simulink model "System_model_discrete"  (R2022a)
settings: Solver=FixedStepDiscrete  StartTime=0.0  StopTime=T_final  FixedStep=T_sample  RelTol=1e-3
values from neighbouring files (symbols this model uses):
  A_bar_d = readmatrix('A_bar_d.csv')    [Run_model_WDS.m]
  B_bar_d = readmatrix('B_bar_d.csv')    [Run_model_WDS.m]
  BDD_thresh = 5    [Run_model_WDS.m]    (also in run_model.m = 0.05)
  C_obsv_d = readmatrix('C_obsv_d.csv')    [Run_model_WDS.m]    (also in run_model.m = C_obsv; run_model_power_system.m = C_obsv)
  D_obsv_d = readmatrix('D_obsv_d.csv')    [Run_model_WDS.m]    (also in run_model.m = D_obsv; run_model_power_system.m = D_obsv)
  l = n_meas    [run_model.m]
  L_obsv = place(A_bar_d.',C_obsv_d.',P).'    [run_model.m]    (also in run_model_power_system.m)
  load_buses = [zeros(n_gen,1); ones(n_bus-n_gen,1)]    [run_model.m]    (also in run_model_power_system.m)
  m = n_meas    [run_model.m]
  max_attack = 1000    [Run_model_WDS.m]
  n = n_states    [run_model.m]
  n_attack = round(attack_percentage*n_meas)    [Run_model_WDS.m]    (also in run_model.m = round(0.2*n_meas))
  n_bus = size(bus,1)    [run_model.m]    (also in run_model_power_system.m)
  n_gen = size(gen,1)    [run_model.m]    (also in run_model_power_system.m)
  n_meas = size(C_obsv_d,1)    [Run_model_WDS.m]    (also in run_model.m = n_gen + n_bus; run_model_power_system.m = n_gen + n_bus)
  n_states = 2*n_gen    [run_model.m]    (also in run_model_power_system.m)
  q0 = ones(m,T)    [run_model.m]
  r_tau = chi2inv(0.1,n_meas)    [Run_model_WDS.m]
  Sigma = diag(sigma)    [Run_model_WDS.m]    (also in run_model.m)
  sigma_inv_k = 1e2*(3 + 2*rand(n_meas,1))    [Run_model_WDS.m]    (also in run_model.m = 1e4*(3 + 2*rand(m,1)); sigma_inv_k.mat = [541957.05841 17086.3156535 20847.4062112 958.936090052 8825)
  Sigma_inv_k = diag(sigma_inv_k)    [Run_model_WDS.m]    (also in run_model.m)
  T = round(2*n_states)    [Run_model_WDS.m]    (also in run_model.m = round(2*n); run_model_power_system.m = 10)
  T_sample = 0.01    [Run_model_WDS.m]    (also in run_model.m; run_model_power_system.m)
  T_start_attack = 0.1*T_final    (= 0.8)    [Run_model_WDS.m]    (also in run_model.m = 1.6; run_model_power_system.m)
  U0 = zeros(n_int,T+1)    [Run_model_WDS.m]    (also in run_model.m = zeros(m,T); run_model_power_system.m)
  x0 = zeros(n_states,1)    [Run_model_WDS.m]    (also in run_model.m; run_model_power_system.m)
  Y0 = zeros(n_meas,T)    [Run_model_WDS.m]    (also in run_model.m = zeros(m,T); run_model_power_system.m)
undefined symbols (not defined in the file or in its folder): G_T, HT, PhiT, sigbuilder_block, T_start_opt, Theta_T
libraries: simulink x5
settings Model: Creator=oanubi  LastModifiedBy=Abelb
settings SolverCC: AlgebraicLoopSolver=TrustRegion
settings DebuggingCC: UnconnectedInputMsg=warning  UnconnectedOutputMsg=warning  UnconnectedLineMsg=warning  SFMachineParentedDataDiag=warning

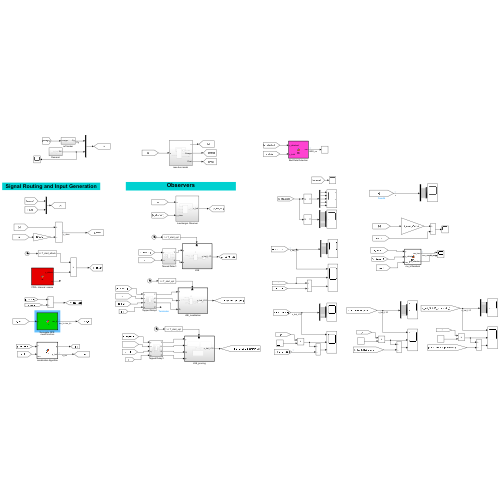
[thumbnail: Simulink's stored preview of the top-level diagram]
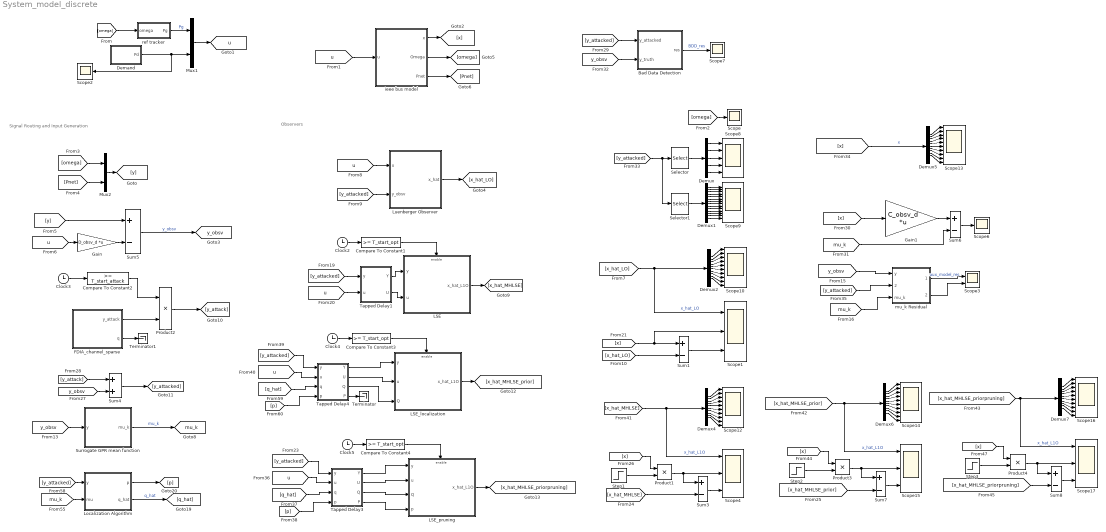
== system System_model_discrete ==
  note: Observers
  note: Signal Routing and Input Generation
  Bad Data Detection : MATLAB Function  TreatAsAtomicUnit=on
  Clock{2..5} (4 alike) : Clock
  Compare To Constant1 : simulink/Logic and Bit Operations/Compare To Constant  relop=>=  const=T_start_opt  OutDataTypeStr=boolean
  Compare To Constant2 : simulink/Logic and Bit Operations/Compare To Constant  relop=>=  const=T_start_attack  OutDataTypeStr=boolean
  Compare To Constant3 : simulink/Logic and Bit Operations/Compare To Constant  relop=>=  const=T_start_opt  OutDataTypeStr=boolean
  Compare To Constant4 : simulink/Logic and Bit Operations/Compare To Constant  relop=>=  const=T_start_opt  OutDataTypeStr=boolean
  Demand : Subsystem
  Demux : Demux  Outputs=n_gen
  Demux1 : Demux  Outputs=n_bus
  Demux{2,4..7} (5 alike) : Demux  Outputs=n_states
  FDIA_channel_sparse : MATLAB Function  TreatAsAtomicUnit=on
  Gain : Gain  Gain=D_obsv_d  Multiplication=Matrix(K*u) (u vector)
  Gain1 : Gain  Gain=C_obsv_d  Multiplication=Matrix(K*u) (u vector)
  LSE : Subsystem
  LSE_localization : Subsystem
  LSE_pruning : Subsystem
  Localization Algorithm : MATLAB Function  TreatAsAtomicUnit=on
  Luenberger Observer : Subsystem
  Mux1 : Mux  Inputs=2
  Mux2 : Mux  Inputs=2
  Product{1..4} (4 alike) : Product
  Scope{,2,6..7} (4 alike) : Scope
  Scope{1,4,15,17} (4 alike) : Scope  NumInputPorts=3
  Scope{10,12..14,16} (5 alike) : Scope  NumInputPorts=10
  Scope3 : Scope  NumInputPorts=2
  Scope8 : Scope  NumInputPorts=5
  Scope9 : Scope  NumInputPorts=14
  Selector : Selector  InputPortWidth=n_meas  IndexOptions=Index vector (dialog)  Indices=1:n_gen  OutputSizes=1
  Selector1 : Selector  InputPortWidth=n_meas  IndexOptions=Index vector (dialog)  Indices=n_gen+1:n_meas  OutputSizes=1
  Step1 : Step  Time=1.5*T*T_sample  SampleTime=0
  Step2 : Step  Time=1.5*T*T_sample  SampleTime=0
  Step3 : Step  Time=1.5*T*T_sample  SampleTime=0
  Sum{1,3,5..8} (6 alike) : Sum  Inputs=+-
  Sum4 : Sum
  Surrogate GPR mean function : MATLAB Function  TreatAsAtomicUnit=on
  Tapped Delay1 : Subsystem
  Tapped Delay3 : Subsystem
  Tapped Delay4 : Subsystem
  Terminator : Terminator
  Terminator1 : Terminator
  ieee bus model : Subsystem
  mu_k Residual : MATLAB Function  TreatAsAtomicUnit=on
  ref tracker : Subsystem
  tag scope: mu_k=global, u=global, y_obsv=global
  wires:
  [u] -> ieee bus model/1(u)
  Demand/1(Pd) -> Scope2/1, Mux1/2
  ref tracker/1(Pg) -> Mux1/1  "Pg"
  Mux1/1 -> [u]
  ieee bus model/2(Omega) -> [omega]
  ieee bus model/1(x) -> [x]
  ieee bus model/3(Pnet) -> [Pnet]
  [omega] -> ref tracker/1(omega)
  [omega] -> Scope/1
  Mux2/1 -> [y]
  [omega] -> Mux2/1
  [Pnet] -> Mux2/2
  [y] -> Sum5/1
  Gain/1 -> Sum5/2
  [u] -> Gain/1
  Sum5/1 -> [y_obsv]  "y_obsv"
  [u] -> Luenberger Observer/1(u)
  [y_attacked] -> Luenberger Observer/2(y_obsv)
  Luenberger Observer/1(x_hat) -> [x_hat_LO]
  [y_obsv] -> Surrogate GPR mean function/1(y)
  Surrogate GPR mean function/1(mu_k) -> [mu_k]  "mu_k"
  [mu_k] -> mu_k Residual/3(mu_k)
  mu_k Residual/1(res_true) -> Scope3/1  "aux_model_res"
  [x_hat_LO] -> Sum1/2
  [x] -> Sum1/1, Scope1/2
  Sum1/1 -> Scope1/3
  LSE/1(x_hat_L1O) -> [x_hat_MHLSE]
  [y_attacked] -> Tapped Delay1/1(y)
  Tapped Delay1/1(Y) -> LSE/1(y)
  [u] -> Tapped Delay1/2(u)
  Clock2/1 -> Compare To Constant1/1
  Tapped Delay1/2(U) -> LSE/2(u)
  Compare To Constant1/1 -> LSE/Enable
  Sum3/1 -> Scope4/3
  [x_hat_MHLSE] -> Sum3/2
  [y_obsv] -> Sum4/2
  Sum4/1 -> [y_attacked]
  [y_attack] -> Sum4/1
  [x] -> Product1/1
  Step1/1 -> Product1/2
  Product1/1 -> Sum3/1, Scope4/2
  Gain1/1 -> Sum6/1
  [x] -> Gain1/1
  [mu_k] -> Sum6/2
  Sum6/1 -> Scope6/1
  [y_obsv] -> mu_k Residual/1(y)
  [y_attacked] -> Bad Data Detection/1(y_attacked)
  Bad Data Detection/1(res) -> Scope7/1  "BDD_res"
  [y_obsv] -> Bad Data Detection/2(y_truth)
  [y_attacked] -> Selector1/1, Selector/1
  Demux/1 -> Scope8/1
  Demux/2 -> Scope8/2
  Demux/3 -> Scope8/3
  Demux/4 -> Scope8/4
  Demux/5 -> Scope8/5
  Selector/1 -> Demux/1
  Selector1/1 -> Demux1/1
  Demux1/5 -> Scope9/5
  Demux1/4 -> Scope9/4
  Demux1/3 -> Scope9/3
  Demux1/2 -> Scope9/2
  Demux1/1 -> Scope9/1
  Demux1/6 -> Scope9/6
  Demux1/7 -> Scope9/7
  Demux1/8 -> Scope9/8
  Demux1/9 -> Scope9/9
  Demux1/10 -> Scope9/10
  Demux1/11 -> Scope9/11
  Demux1/12 -> Scope9/12
  Demux1/13 -> Scope9/13
  Demux1/14 -> Scope9/14
  [x_hat_LO] -> Demux2/1, Scope1/1  "x_hat_LO"
  Demux2/1 -> Scope10/1
  Demux2/2 -> Scope10/2
  Demux2/3 -> Scope10/3
  Demux2/4 -> Scope10/4
  Demux2/5 -> Scope10/5
  Demux2/6 -> Scope10/6
  Demux2/7 -> Scope10/7
  Demux2/8 -> Scope10/8
  Demux2/9 -> Scope10/9
  Demux2/10 -> Scope10/10
  Demux4/9 -> Scope12/9
  Demux4/1 -> Scope12/1
  Demux4/7 -> Scope12/7
  Demux4/2 -> Scope12/2
  Demux4/4 -> Scope12/4
  Demux4/5 -> Scope12/5
  Demux4/10 -> Scope12/10
  Demux4/8 -> Scope12/8
  Demux4/3 -> Scope12/3
  [x_hat_MHLSE] -> Demux4/1, Scope4/1  "x_hat_L1O"
  Demux4/6 -> Scope12/6
  [x] -> Demux5/1  "x"
  Demux5/10 -> Scope13/10
  Demux5/6 -> Scope13/6
  Demux5/8 -> Scope13/8
  Demux5/5 -> Scope13/5
  Demux5/3 -> Scope13/3
  Demux5/7 -> Scope13/7
  Demux5/2 -> Scope13/2
  Demux5/1 -> Scope13/1
  Demux5/4 -> Scope13/4
  Demux5/9 -> Scope13/9
  Product2/1 -> [y_attack]
  FDIA_channel_sparse/1(y_attack) -> Product2/2
  Compare To Constant2/1 -> Product2/1
  Clock3/1 -> Compare To Constant2/1
  mu_k Residual/2(res_attacked) -> Scope3/2
  [y_attacked] -> mu_k Residual/2(y_attacked)
  [y_attacked] -> Localization Algorithm/1(y)
  Localization Algorithm/1(p) -> [p]
  [mu_k] -> Localization Algorithm/2(mu)
  Localization Algorithm/2(q_hat) -> [q_hat]  "q_hat"
  Clock4/1 -> Compare To Constant3/1
  Compare To Constant3/1 -> LSE_localization/Enable
  LSE_localization/1(x_hat_L1O) -> [x_hat_MHLSE_prior]
  Tapped Delay4/2(U) -> LSE_localization/2(u)
  [y_attacked] -> Tapped Delay4/1(y)
  Tapped Delay4/3(Q) -> LSE_localization/3(Q)
  [u] -> Tapped Delay4/2(u)
  Tapped Delay4/1(Y) -> LSE_localization/1(y)
  [q_hat] -> Tapped Delay4/3(q)
  [p] -> Tapped Delay4/4(p)
  LSE_pruning/1(x_hat_L1O) -> [x_hat_MHLSE_priorpruning]
  Compare To Constant4/1 -> LSE_pruning/Enable
  Clock5/1 -> Compare To Constant4/1
  Tapped Delay3/1(Y) -> LSE_pruning/1(y)
  [q_hat] -> Tapped Delay3/3(q)
  [u] -> Tapped Delay3/2(u)
  [y_attacked] -> Tapped Delay3/1(y)
  Tapped Delay3/4(P) -> LSE_pruning/4(p)
  Tapped Delay3/2(U) -> LSE_pruning/2(u)
  [p] -> Tapped Delay3/4(p)
  Tapped Delay3/3(Q) -> LSE_pruning/3(Q)
  Tapped Delay4/4(P) -> Terminator/1
  [x_hat_MHLSE_prior] -> Sum7/2
  [x_hat_MHLSE_prior] -> Demux6/1, Scope15/1  "x_hat_L1O"
  Demux6/6 -> Scope14/6
  Demux6/3 -> Scope14/3
  Demux6/7 -> Scope14/7
  Demux6/8 -> Scope14/8
  Demux6/4 -> Scope14/4
  Demux6/1 -> Scope14/1
  Demux6/5 -> Scope14/5
  Product3/1 -> Sum7/1, Scope15/2
  Demux6/9 -> Scope14/9
  [x] -> Product3/1
  Step2/1 -> Product3/2
  Demux6/2 -> Scope14/2
  Demux6/10 -> Scope14/10
  Sum7/1 -> Scope15/3
  Sum8/1 -> Scope17/3
  Demux7/10 -> Scope16/10
  Demux7/8 -> Scope16/8
  Demux7/9 -> Scope16/9
  Demux7/2 -> Scope16/2
  [x] -> Product4/1
  Demux7/7 -> Scope16/7
  Demux7/3 -> Scope16/3
  Step3/1 -> Product4/2
  Product4/1 -> Sum8/1, Scope17/2
  Demux7/5 -> Scope16/5
  Demux7/1 -> Scope16/1
  [x_hat_MHLSE_priorpruning] -> Demux7/1, Scope17/1  "x_hat_L1O"
  [x_hat_MHLSE_priorpruning] -> Sum8/2
  Demux7/6 -> Scope16/6
  Demux7/4 -> Scope16/4
  FDIA_channel_sparse/2(q) -> Terminator1/1

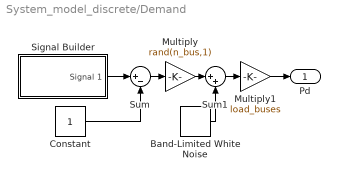
== system System_model_discrete/Demand ==
  Band-Limited White Noise : simulink/Sources/Band-Limited White Noise  Cov=1e-8  Ts=0.1  seed=[23341]
  Constant : Constant
  Multiply : Gain  Gain=rand(n_bus,1)
  Multiply1 : Gain  Gain=load_buses
  Signal Builder : Subsystem  Tag=STV Subsys  LoadFcn=sigbuilder_block('load');  StartFcn=sigbuilder_block('start');  StopFcn=sigbuilder_block('stop');  ClipboardFcn=sigbuilder_block('clipboard');  mask(Sigbuilder block){tuvar=[0:10]}
      mask help: Simulink:masks:SigbuilderBlock_MD
      mask init:
      | if ~strcmp(get_param(bdroot(gcbh),'SimulationStatus'),'stopped') tuvar = sigbuilder_block('maskInit'); end
      settings: CopyFcn=sigbuilder_block('copy');  DeleteFcn=sigbuilder_block('delete');  ModelCloseFcn=sigbuilder_block('modelClose');  PreSaveFcn=sigbuilder_block('preSave');  PauseFcn=sigbuilder_block('pause');  ContinueFcn=sigbuilder_block('continue');  NameChangeFcn=sigbuilder_block('namechange');  OpenFcn=sigbuilder_block('open',[439.2 145.2 550.2 399.9 ]);  CloseFcn=sigbuilder_block('close');
      mask Display: plot(0, 0, 100, 100,[2, 2, 32, 32, 2], [68, 8, 8, 68, 68],[32, 2], [38, 38], [32, 19, 2],[53, 60, 44], [32, 17, 17, 2],[16, 16, 31, 31]);txt = getActiveGroup(gcbh);text(2, 100, txt,'verticalAlignment', 'top');
  Sum : Sum  Inputs=|+-
  Sum1 : Sum  Inputs=|++
  Pd : Outport
  wires:
  Sum/1 -> Multiply/1
  Signal Builder/1(Signal 1) -> Sum/1
  Constant/1 -> Sum/2
  Multiply/1 -> Sum1/1
  Band-Limited White Noise/1 -> Sum1/2
  Sum1/1 -> Multiply1/1
  Multiply1/1 -> Pd/1

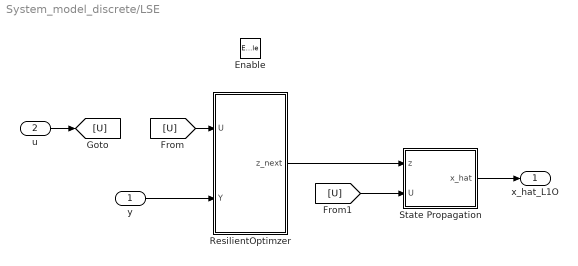
== system System_model_discrete/LSE ==
  y : Inport
  u : Inport  Port=2
  Enable : EnablePort
  ResilientOptimzer : MATLAB Function  TreatAsAtomicUnit=on
  State Propagation : MATLAB Function  TreatAsAtomicUnit=on
  x_hat_L1O : Outport
  wires:
  ResilientOptimzer/1(z_next) -> State Propagation/1(z)
  u/1 -> [U]
  y/1 -> ResilientOptimzer/2(Y)
  [U] -> ResilientOptimzer/1(U)
  [U] -> State Propagation/2(U)
  State Propagation/1(x_hat) -> x_hat_L1O/1

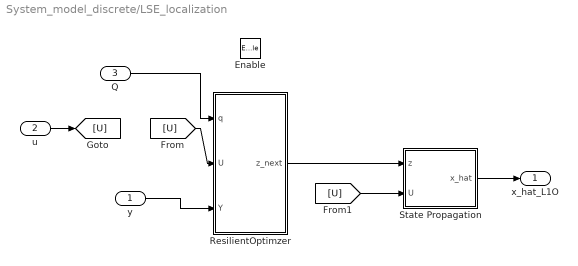
== system System_model_discrete/LSE_localization ==
  y : Inport
  u : Inport  Port=2
  Q : Inport  Port=3
  Enable : EnablePort
  ResilientOptimzer : MATLAB Function  TreatAsAtomicUnit=on
  State Propagation : MATLAB Function  TreatAsAtomicUnit=on
  x_hat_L1O : Outport
  wires:
  ResilientOptimzer/1(z_next) -> State Propagation/1(z)
  u/1 -> [U]
  y/1 -> ResilientOptimzer/3(Y)
  [U] -> ResilientOptimzer/2(U)
  [U] -> State Propagation/2(U)
  State Propagation/1(x_hat) -> x_hat_L1O/1
  Q/1 -> ResilientOptimzer/1(q)

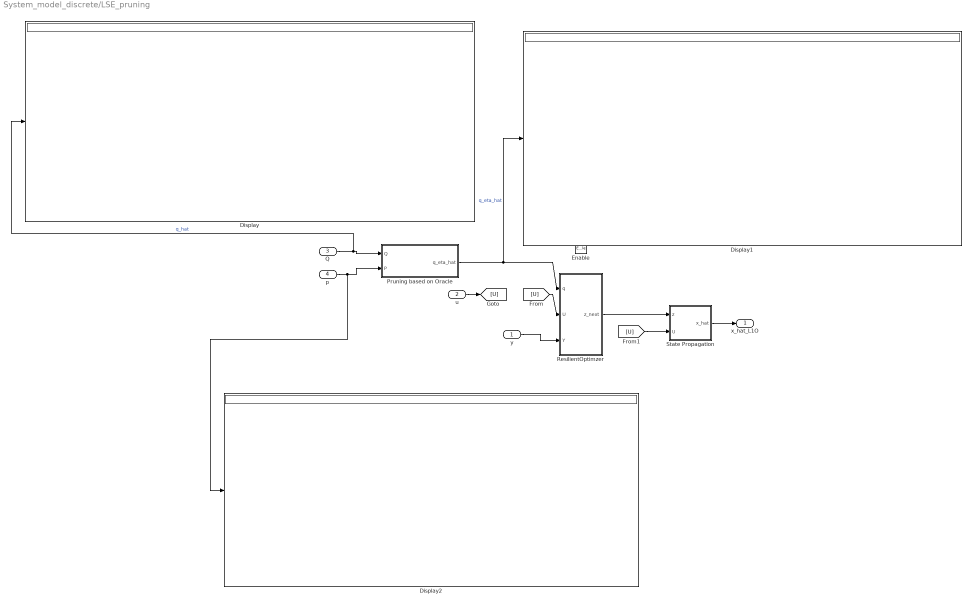
== system System_model_discrete/LSE_pruning ==
  y : Inport
  u : Inport  Port=2
  Q : Inport  Port=3
  p : Inport  Port=4
  Enable : EnablePort
  Display : Display
  Display1 : Display
  Display2 : Display
  Pruning based on Oracle : MATLAB Function  TreatAsAtomicUnit=on
  ResilientOptimzer : MATLAB Function  TreatAsAtomicUnit=on
  State Propagation : MATLAB Function  TreatAsAtomicUnit=on
  x_hat_L1O : Outport
  wires:
  ResilientOptimzer/1(z_next) -> State Propagation/1(z)
  u/1 -> [U]
  y/1 -> ResilientOptimzer/3(Y)
  [U] -> ResilientOptimzer/2(U)
  [U] -> State Propagation/2(U)
  State Propagation/1(x_hat) -> x_hat_L1O/1
  Q/1 -> Display/1, Pruning based on Oracle/1(Q)  "q_hat"
  Pruning based on Oracle/1(q_eta_hat) -> Display1/1, ResilientOptimzer/1(q)  "q_eta_hat"
  p/1 -> Display2/1, Pruning based on Oracle/2(P)

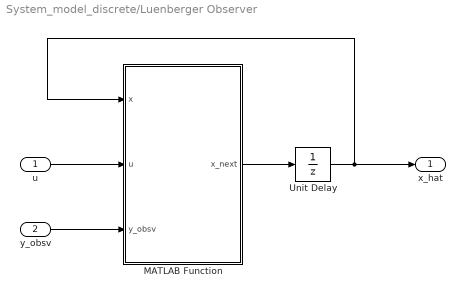
== system System_model_discrete/Luenberger Observer ==
  u : Inport
  y_obsv : Inport  Port=2
  MATLAB Function : MATLAB Function  TreatAsAtomicUnit=on
  Unit Delay : UnitDelay  InitialCondition=zeros(n_states,1)  SampleTime=-1  HasFrameUpgradeWarning=on
  x_hat : Outport
  wires:
  MATLAB Function/1(x_next) -> Unit Delay/1
  Unit Delay/1 -> x_hat/1, MATLAB Function/1(x)
  u/1 -> MATLAB Function/2(u)
  y_obsv/1 -> MATLAB Function/3(y_obsv)

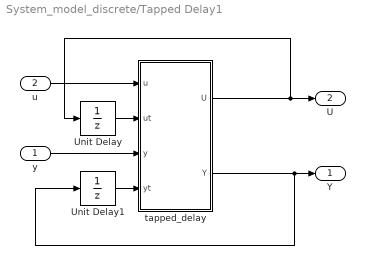
== system System_model_discrete/Tapped Delay1 ==
  y : Inport
  u : Inport  Port=2
  Unit Delay : UnitDelay  InitialCondition=U0  SampleTime=-1  HasFrameUpgradeWarning=on
  Unit Delay1 : UnitDelay  InitialCondition=Y0  SampleTime=-1  HasFrameUpgradeWarning=on
  tapped_delay : MATLAB Function  TreatAsAtomicUnit=on
  Y : Outport
  U : Outport  Port=2
  wires:
  u/1 -> tapped_delay/1(u)
  y/1 -> tapped_delay/3(y)
  tapped_delay/1(U) -> Unit Delay/1, U/1
  tapped_delay/2(Y) -> Unit Delay1/1, Y/1
  Unit Delay/1 -> tapped_delay/2(ut)
  Unit Delay1/1 -> tapped_delay/4(yt)

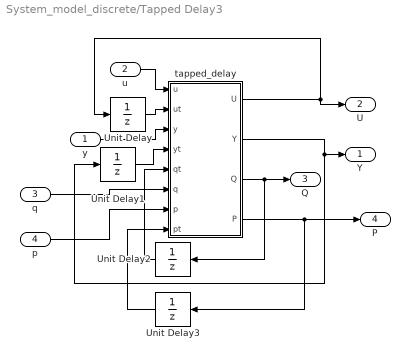
== system System_model_discrete/Tapped Delay3 ==
  y : Inport
  u : Inport  Port=2
  q : Inport  Port=3
  p : Inport  Port=4
  Unit Delay : UnitDelay  InitialCondition=U0  SampleTime=-1  HasFrameUpgradeWarning=on
  Unit Delay1 : UnitDelay  InitialCondition=Y0  SampleTime=-1  HasFrameUpgradeWarning=on
  Unit Delay2 : UnitDelay  InitialCondition=q0  SampleTime=-1  HasFrameUpgradeWarning=on
  Unit Delay3 : UnitDelay  InitialCondition=q0  SampleTime=-1  HasFrameUpgradeWarning=on
  tapped_delay : MATLAB Function  TreatAsAtomicUnit=on
  Y : Outport
  U : Outport  Port=2
  Q : Outport  Port=3
  P : Outport  Port=4
  wires:
  u/1 -> tapped_delay/1(u)
  y/1 -> tapped_delay/3(y)
  tapped_delay/1(U) -> U/1, Unit Delay/1
  tapped_delay/2(Y) -> Unit Delay1/1, Y/1
  Unit Delay/1 -> tapped_delay/2(ut)
  Unit Delay1/1 -> tapped_delay/4(yt)
  tapped_delay/3(Q) -> Unit Delay2/1, Q/1
  Unit Delay2/1 -> tapped_delay/5(qt)
  q/1 -> tapped_delay/6(q)
  p/1 -> tapped_delay/7(p)
  tapped_delay/4(P) -> Unit Delay3/1, P/1
  Unit Delay3/1 -> tapped_delay/8(pt)

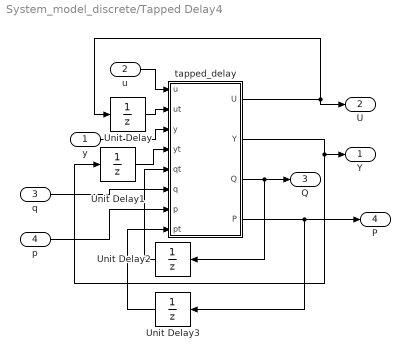
== system System_model_discrete/Tapped Delay4 ==
  y : Inport
  u : Inport  Port=2
  q : Inport  Port=3
  p : Inport  Port=4
  Unit Delay : UnitDelay  InitialCondition=U0  SampleTime=-1  HasFrameUpgradeWarning=on
  Unit Delay1 : UnitDelay  InitialCondition=Y0  SampleTime=-1  HasFrameUpgradeWarning=on
  Unit Delay2 : UnitDelay  InitialCondition=q0  SampleTime=-1  HasFrameUpgradeWarning=on
  Unit Delay3 : UnitDelay  InitialCondition=q0  SampleTime=-1  HasFrameUpgradeWarning=on
  tapped_delay : MATLAB Function  TreatAsAtomicUnit=on
  Y : Outport
  U : Outport  Port=2
  Q : Outport  Port=3
  P : Outport  Port=4
  wires:
  u/1 -> tapped_delay/1(u)
  y/1 -> tapped_delay/3(y)
  tapped_delay/1(U) -> U/1, Unit Delay/1
  tapped_delay/2(Y) -> Unit Delay1/1, Y/1
  Unit Delay/1 -> tapped_delay/2(ut)
  Unit Delay1/1 -> tapped_delay/4(yt)
  tapped_delay/3(Q) -> Unit Delay2/1, Q/1
  Unit Delay2/1 -> tapped_delay/5(qt)
  q/1 -> tapped_delay/6(q)
  p/1 -> tapped_delay/7(p)
  tapped_delay/4(P) -> Unit Delay3/1, P/1
  Unit Delay3/1 -> tapped_delay/8(pt)

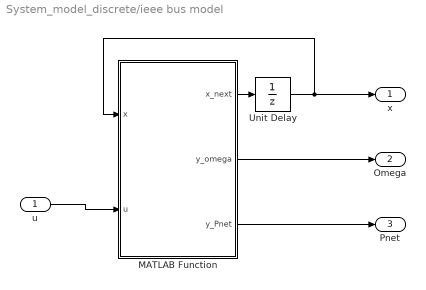
== system System_model_discrete/ieee bus model ==
  u : Inport
  MATLAB Function : MATLAB Function  TreatAsAtomicUnit=on
  Unit Delay : UnitDelay  InitialCondition=x0  SampleTime=-1  HasFrameUpgradeWarning=on
  x : Outport
  Omega : Outport  Port=2
  Pnet : Outport  Port=3
  wires:
  MATLAB Function/1(x_next) -> Unit Delay/1
  Unit Delay/1 -> x/1, MATLAB Function/1(x)
  u/1 -> MATLAB Function/2(u)
  MATLAB Function/2(y_omega) -> Omega/1
  MATLAB Function/3(y_Pnet) -> Pnet/1

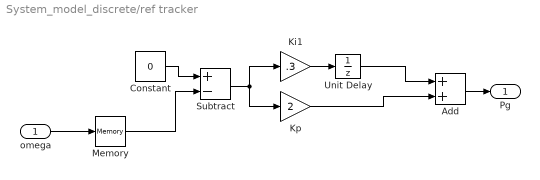
== system System_model_discrete/ref tracker ==
  omega : Inport
  Add : Sum
  Constant : Constant  Value=0
  Ki1 : Gain  Gain=.3
  Kp : Gain  Gain=2
  Memory : Memory  InitialCondition=zeros(n_gen,1)
  Subtract : Sum  Inputs=+-
  Unit Delay : UnitDelay  InitialCondition=zeros(n_gen,1)  SampleTime=-1  HasFrameUpgradeWarning=on
  Pg : Outport
  wires:
  Kp/1 -> Add/2
  Unit Delay/1 -> Add/1
  Add/1 -> Pg/1
  Constant/1 -> Subtract/1
  Subtract/1 -> Ki1/1, Kp/1
  Ki1/1 -> Unit Delay/1
  Memory/1 -> Subtract/2
  omega/1 -> Memory/1

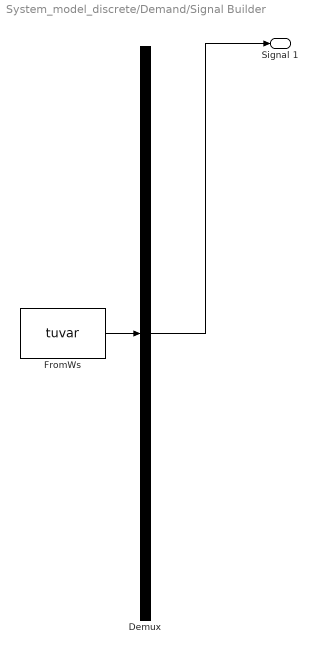
== system System_model_discrete/Demand/Signal Builder ==
  Demux : Demux  Tag=STV Demux  Outputs=1
      settings: DisplayOption=none
  FromWs : FromWorkspace  Tag=STV FromWs  VariableName=tuvar
      SigBuilderData=|
      | common.afterFinalStr = 'Extrapolate'
      | common.sampleTime = 0
      | dataSet.timeRange = [0 10]
      | dataSet.name = 'Group 1'
      | sbobj.Groups.Name = 'Group 1'
      | sbobj.Groups.Signals.Name = 'Signal 1'
      | sbobj.Groups.Signals.XData = [0 0.46 1.5 2.5 4 5 6 7 10]
      | sbobj.Groups.Signals.YData = [1 1.106 1.2 1.2 0.8 0.8 1 1 1]
  Signal 1 : Outport  Tag=STV Outport
  wires:
  Demux/1 -> Signal 1/1
  FromWs/1 -> Demux/1

== matlab function System_model_discrete/FDIA_channel_sparse ==
  data: n_attack parameter; y_attack output; n_meas parameter; C_obsv_d parameter; max_attack parameter; BDD_thresh parameter; q output
function [y_attack,q] = fcn(n_attack,n_meas,C_obsv_d,max_attack, BDD_thresh)

%% Measurement Channel Attack
%  Assumptions:
%  1. The attacker knows the actual measurement
%  2. The attacker can only corrupt upto n_attack measurements
%  3. The attacker knows the BDD theshold

attack_idx = randi(n_meas,n_attack,1);
y_attack   = gen_attack_channel(C_obsv_d, max_attack,attack_idx,0.75*BDD_thresh);
                                                        % NOTE THE .75
                                                        % Used
                                                        % conservatively
q = ones(n_meas,1);
q(attack_idx) = 0;

== matlab function System_model_discrete/Bad Data Detection ==
  data: y_attacked input; y_truth input; res output; U2 parameter
function res = fcn(y_attacked,y_truth,U2)

res = [norm(U2.'*y_attacked,2);
       norm(U2.'*y_truth,2)];

== matlab function System_model_discrete/LSE_localization/ResilientOptimzer ==
  data: q input; z_next output; U input; Y input; HT parameter; PhiT parameter; n_states parameter; l parameter; T parameter
function z_next  = fcn(q,U,Y, HT, PhiT, n_states,l,T)
u_local = zeros(l,T-1);
u_local(:,:) = U(:,1:end-1);
% vectorized
u = u_local(:);
y = Y(:);

coder.extrinsic('solver_call_oracle')
z_next = zeros(n_states,1);
z_next(:) = solver_call_oracle(y,u,HT,PhiT,q);

== matlab function System_model_discrete/LSE_localization/State Propagation ==
  data: z input; x_hat output; U input; Theta_T parameter; G_T parameter; n parameter; T parameter; l parameter
function x_hat = fcn(z,U,Theta_T, G_T,n,T,l)
% x_hat = fcn(z,U,PhiT, HT,n_states)
% Propagates the estimated intial state to the current time
u_local = zeros(l,T-1);
u_local(:,:) = U(:,1:end-1);


% State propagation
x_hat = Theta_T*z(1:n) + G_T*u_local(:);

== matlab function System_model_discrete/LSE_pruning/Pruning based on Oracle ==
  data: Q input; q_eta_hat output; P input
function q_eta_hat = fcn(Q,P)

q = Q(:);
p = P(:);

coder.extrinsic('pruning_algorithm')
q_eta_hat = ones(size(q));
q_eta_hat(:) = pruning_algorithm(q,p);

== matlab function System_model_discrete/LSE_pruning/ResilientOptimzer ==
  data: q input; z_next output; U input; Y input; HT parameter; PhiT parameter; n_states parameter; l parameter; T parameter
function z_next  = fcn(q,U,Y, HT, PhiT, n_states,l,T)
u_local = zeros(l,T-1);
u_local(:,:) = U(:,1:end-1);
% vectorized
u = u_local(:);
y = Y(:);

coder.extrinsic('solver_call_oracle')
z_next = zeros(n_states,1);
z_next(:) = solver_call_oracle(y,u,HT,PhiT,q);

== matlab function System_model_discrete/LSE_pruning/State Propagation ==
  data: z input; x_hat output; U input; Theta_T parameter; G_T parameter; n parameter; T parameter; l parameter
function x_hat = fcn(z,U,Theta_T, G_T,n,T,l)
% x_hat = fcn(z,U,PhiT, HT,n_states)
% Propagates the estimated intial state to the current time
u_local = zeros(l,T-1);
u_local(:,:) = U(:,1:end-1);


% State propagation
x_hat = Theta_T*z(1:n) + G_T*u_local(:);

== matlab function System_model_discrete/Tapped Delay4/tapped_delay ==
  data: u input; U output; ut input; y input; yt input; Y output; qt input; Q output; q input; p input; pt input; P output
function [U,Y,Q,P] = fcn(u,ut,y,yt,qt, q, p,pt)
%% tapped_delay_array
% shift columns from tapped matrix to the left and appends most recent
% vector to the last column
%%% input
ut(:,1:end-1) = ut(:,2:end);
ut(:,end) = u;
U = ut;
%%% output
yt(:,1:end-1) = yt(:,2:end);
yt(:,end) = y;
Y = yt;
%%% attack
qt(:,1:end-1) = qt(:,2:end);
qt(:,end) = q;
Q = qt;
%%% confidence
pt(:,1:end-1) = pt(:,2:end);
pt(:,end) = p;
P = pt;

== matlab function System_model_discrete/Luenberger Observer/MATLAB Function ==
  data: x input; x_next output; u input; y_obsv input; L_obsv parameter; A_bar_d parameter; C_obsv_d parameter; B_bar_d parameter
function x_next  = fcn(x,u,y_obsv,L_obsv,A_bar_d,C_obsv_d,B_bar_d)
% Discrete state-space model for system

x_next = A_bar_d*x + B_bar_d*u + L_obsv*(y_obsv - C_obsv_d*x);

== matlab function System_model_discrete/Tapped Delay3/tapped_delay ==
  data: u input; U output; ut input; y input; yt input; Y output; qt input; Q output; q input; p input; pt input; P output
function [U,Y,Q,P] = fcn(u,ut,y,yt,qt, q, p,pt)
%% tapped_delay_array
% shift columns from tapped matrix to the left and appends most recent
% vector to the last column
%%% input
ut(:,1:end-1) = ut(:,2:end);
ut(:,end) = u;
U = ut;
%%% output
yt(:,1:end-1) = yt(:,2:end);
yt(:,end) = y;
Y = yt;
%%% attack
qt(:,1:end-1) = qt(:,2:end);
qt(:,end) = q;
Q = qt;
%%% confidence
pt(:,1:end-1) = pt(:,2:end);
pt(:,end) = p;
P = pt;

== matlab function System_model_discrete/Localization Algorithm ==
  data: p output; y input; q_hat output; mu input; Sigma parameter; n_meas parameter
function [p, q_hat] = fcn(y,mu,Sigma, n_meas)

%% calculate probability
z = (y - mu)./diag(Sigma);
p = 2*(ones(n_meas,1)-normcdf(abs(z)));

%% support prior and corresponding confidence
% q_hat = zeros(n_meas,1);
% q_hat(p >= 0.5) = 1;
q_hat = double(p>=0.5);

== matlab function System_model_discrete/ieee bus model/MATLAB Function ==
  data: x input; x_next output; u input; y_omega output; A_bar_d parameter; C_obsv_d parameter; B_bar_d parameter; D_obsv_d parameter; n_gen parameter; n_bus parameter; y_Pnet output
function [x_next,y_omega,y_Pnet] = fcn(x,u,A_bar_d,C_obsv_d,B_bar_d,D_obsv_d,n_gen, n_bus)
% Discrete state-space model for system

x_next = A_bar_d*x + B_bar_d*u;

y = C_obsv_d*x + D_obsv_d*u;

y_omega = y(1:n_gen);
y_Pnet = y(n_gen+1:n_bus+n_gen);

== matlab function System_model_discrete/mu_k Residual ==
  data: y input; y_attacked input; res_true output; mu_k input; Sigma_inv_k parameter; r_tau parameter; res_attacked output
function [res_true,res_attacked] = fcn(y,y_attacked,mu_k,Sigma_inv_k, r_tau)

res_true = r_tau - (y-mu_k).'*Sigma_inv_k*(y-mu_k);
res_attacked = r_tau - (y_attacked-mu_k).'*Sigma_inv_k*(y_attacked-mu_k);

== matlab function System_model_discrete/Surrogate GPR mean function ==
  data: y input; mu_k output; sigma_inv_k parameter; r_tau parameter; m parameter
function mu_k = fcn(y,sigma_inv_k, r_tau,m)
% Prunes a random vector to find mu_k so that ||y-mu_k||_Sigma_inv_k <= r_tau

% first: random vector, secomd: normalize
y_rand = rand(m,1);
y_rand = sqrt(r_tau/max(sigma_inv_k))/norm(y_rand)*y_rand;

% create mu_k from y
mu_k = y - y_rand;

% mu_k = (U_y_1*U_y_1.')*y;

== matlab function System_model_discrete/LSE/ResilientOptimzer ==
  data: z_next output; U input; Y input; HT parameter; PhiT parameter; n_states parameter; l parameter; T parameter
function z_next  = fcn(U,Y, HT, PhiT, n_states,l,T)
u_local = zeros(l,T-1);
u_local(:,:) = U(:,1:end-1);
% vectorized
u = u_local(:);
y = Y(:);

coder.extrinsic('solver_call_unc')
z_next = zeros(n_states,1);
z_next(:) = solver_call_unc(y,u,HT,PhiT);

== matlab function System_model_discrete/LSE/State Propagation ==
  data: z input; x_hat output; U input; Theta_T parameter; G_T parameter; n parameter; T parameter; l parameter
function x_hat = fcn(z,U,Theta_T, G_T,n,T,l)
% x_hat = fcn(z,U,PhiT, HT,n_states)
% Propagates the estimated intial state to the current time
u_local = zeros(l,T-1);
u_local(:,:) = U(:,1:end-1);


% State propagation
x_hat = Theta_T*z(1:n) + G_T*u_local(:);

== matlab function System_model_discrete/Tapped Delay1/tapped_delay ==
  data: u input; U output; ut input; y input; yt input; Y output
function [U,Y] = fcn(u,ut,y,yt)
%% tapped_delay_array
% shift columns from tapped matrix to the left and appends most recent
% vector to the last column
%%% input
ut(:,1:end-1) = ut(:,2:end);
ut(:,end) = u;
U = ut;
%%% output
yt(:,1:end-1) = yt(:,2:end);
yt(:,end) = y;
Y = yt;
